simulink model "SPM_trial_5_simulink"  (R2023a)
settings: Solver=VariableStepAuto  StartTime=0.0  StopTime=500  RelTol=1e-3
values from neighbouring files (symbols this model uses):
  x_neg = 0:dx_n:del_n    [Generate_Amat_Electrolyte.m]
  x_pos = del_n+del_s:dx_p:del_n+del_s+del_p    [Generate_Amat_Electrolyte.m]
  x_sep = del_n:dx_s:del_n+del_s    [Generate_Amat_Electrolyte.m]
undefined symbols (not defined in the file or in its folder): CC, cs_init_n, cs_init_p, I, Iin, Ilim, Kaw, KI, nn, np, ns, sw, Vlim, Vmax
libraries: nesl_utility x16, fl_lib x4
settings Model: Creator=YASH PATHAK  LastModifiedBy=siegeljb
settings ModelReferenceCC: EnableRefExpFcnMdlSchedulingChecks=on

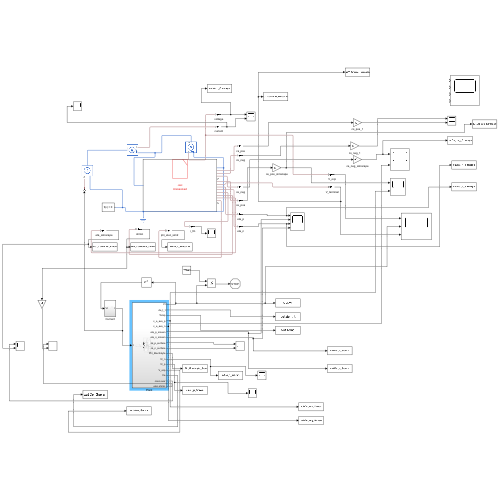
[thumbnail: Simulink's stored preview of the top-level diagram]
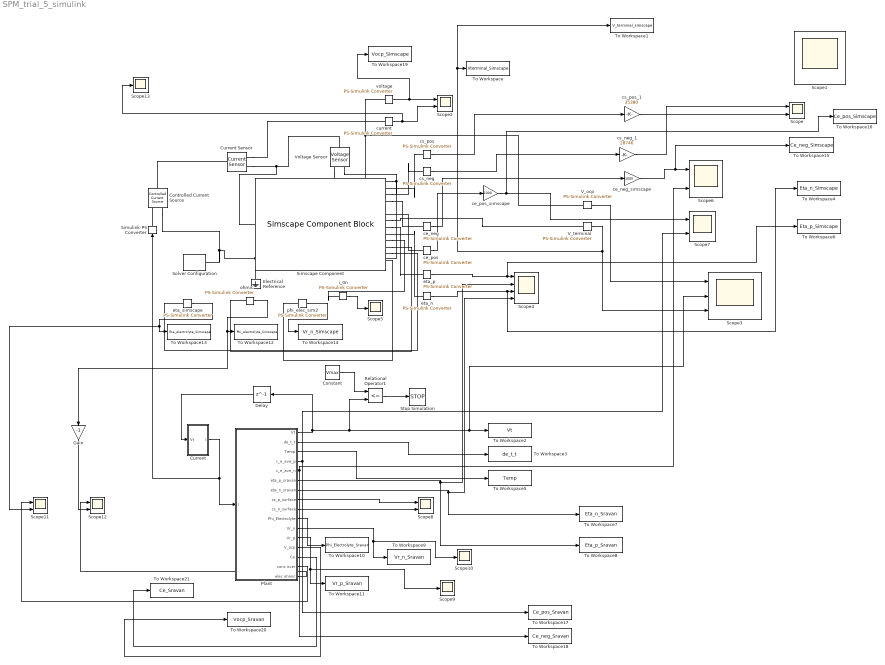
== system SPM_trial_5_simulink ==
  Constant : Constant  Value=Vmax
  Controlled Current Source : fl_lib/Electrical/Electrical Sources/Controlled Current Source
  Current : Subsystem
  Current Sensor : fl_lib/Electrical/Electrical Sensors/Current Sensor
  Delay : Delay  DelayLength=1
  Electrical Reference : fl_lib/Electrical/Electrical Elements/Electrical Reference
  Gain : Gain  Gain=-1
  Plant : Subsystem
  Relational Operator1 : RelationalOperator  Operator=<=  OutDataTypeStr=boolean  RndMeth=Simplest  InputSameDT=off
  Scope{,2,6..8,11..12} (7 alike) : Scope  NumInputPorts=2
  Scope1 : Scope  NumInputPorts=4
  Scope{5,9..10,13} (4 alike) : Scope
  Scope3 : Scope  NumInputPorts=3
  Scope4 : Scope  NumInputPorts=4
  Simscape Component : SimscapeComponentBlock  SourceFile=SPM_Trial_4_2  ComponentPath=SPM_Trial_4_2  ComponentVariants="[\"SPM_Trial_4_2\"]"  ComponentVariantNames="[\"SPM_Trial_4_2\"]"  ClassName=SPM_Trial_4_2  SchemaVersion=1  nr=50  nn=50  ns=25  np=50  Rp=3.5e-06 m  Rn=2.5e-06 m  Ds_p=8e-15 m^2/s  Ds_n=5e-15 m^2/s  D_e=5.35e-10 m^2/s  D_e1=5.35e-10  SOC_0=0.1  brugg=1.5  t_plus=0.38  tf=0.62  ce_init=1000 mol/m^3  ce_init_unitless=1000  kappa=1.3 S/m  k0_n=1.061e-6 / 96485  k0_p=4.824e-6 / 96485  kt_n=1 * 0.0250 V*m^2/A  kt_p=0 * 300e-4 V*m^2/A  x100_percent_n=0.8292  x0_percent_n=3.5506e-04  y0_percent_p=0.8941  y100_percent_p=0.0335  del_p=6.7e-05 m  del_n=6.2e-05 m  del_s=1.2e-05 m  del_p1=6.7e-05  del_n1=6.2e-05  del_s1=1.2e-05  cs_max_p=35380 mol/m^3  cs_max_p_unitless=35380  cs_max_n=28746 mol/m^3  cs_max_n_unitless=28746  epsilon_e_p=0.3  epsilon_e_n=0.3  epsilon_e_s=0.4  Active_Area=0.205 m^2  Faradays=96485 C/mol  T=273.15 + 25  R=8.3145  Cap_n=6.0272 C  Cap_p=5.8050 C  i_specify=off  i_priority=None  i=0 A  i_nominal_specify=off  i_nominal_unit=A  i_nominal_value=1  v_specify=off  v_priority=None  v=0 V  v_nominal_specify=off  v_nominal_unit=V  v_nominal_value=1  UP_specify=off  UP_priority=None  UP=0  UP_nominal_specify=off  UP_nominal_unit=1  UP_nominal_value=1  UN_specify=off  UN_priority=None  UN=0  UN_nominal_specify=off  UN_nominal_unit=1  UN_nominal_value=1  V_ocp_specify=off  V_ocp_priority=None  V_ocp=0  V_ocp_nominal_specify=off  V_ocp_nominal_unit=1  V_ocp_nominal_value=1  j_n_specify=off  j_n_priority=None  j_n=0  j_n_nominal_specify=off  j_n_nominal_unit=1  j_n_nominal_value=1  j_p_specify=off  j_p_priority=None  j_p=0  j_p_nominal_specify=off  j_p_nominal_unit=1  j_p_nominal_value=1  i0_p_specify=off  i0_p_priority=None  i0_p=0  i0_p_nominal_specify=off  i0_p_nominal_unit=1  i0_p_nominal_value=1  Vr_p_specify=off  Vr_p_priority=None  Vr_p=0  Vr_p_nominal_specify=off  Vr_p_nominal_unit=1  Vr_p_nominal_value=1  x_specify=off  x_priority=None  x=0  x_nominal_specify=off  x_nominal_unit=1  x_nominal_value=1  y_specify=off  y_priority=None  y=0  y_nominal_specify=off  y_nominal_unit=1  y_nominal_value=1
      settings: CopyFcn=simscape.engine.sli.internal.componentblockcallback(gcbh,'COPY')  PreCopyFcn=simscape.engine.sli.internal.componentblockcallback(gcbh,'PRECOPY')  PreDeleteFcn=simscape.engine.sli.internal.componentblockcallback(gcbh,'PREDELETE')  InternalSimscapePortConfiguration="{\"Bottom\":[],\"Left\":[{\"id\":\"p\",\"label\":\"+\",\"type\":\"foundation.electrical.electrical\"}],\"Right\":[{\"id\":\"n\",\"label\":\"-\",\"type\":\"foundation.electrical.electrical\"},{\"id\":\"cs_surf_p\",\"label\":\"cs_surf_p\",\"type\":\"output\"},{\"id\":\"cs_surf_n\",\"label\":\"cs_surf_n\",\"type\":\"output\"},{\"id\":\"ce_ave_n\",\"label\":\"ce_ave_n\",\"type\":\"output\"},{\"id\":\"ce_ave_s\",\"label\":\"ce_ave_s\",\"type\":\"output\"},{\"id\":\"ce_ave_p\",\"label\":\"ce_ave_p\",\"type\":\"output\"},{\"id\":\"V_terminal\",\"label\":\"V_terminal\",\"type\":\"output\"},{\"id\":\"eta_p\",\"label\":\"eta_p\",\"type\":\"output\"},{\"id\":\"eta_n\",\"label\":\"eta_n\",\"type\":\"output\"},{\"id\":\"i0_n\",\"label\":\"i0_n\",\"type\":\"output\"},{\"id\":\"phi_electrolyte\",\"label\":\"phi_electrolyte\",\"type\":\"output\"},{\"id\":\"eta_c\",\"label\":\"eta_c\",\"type\":\"output\"},{\"id\":\"Vr_n\",\"label\":\"Vr_n\",\"type\":\"output\"},{\"id\":\"ce_1\",\"label\":\"ce_1\",\"type\":\"output\"}],\"Top\":[]}"
      mask Type: Two-port electrical component
      mask Display: color('red');plot([0 1 1 0 0],[0 0 1 1 0]);plot([0.7,1],[1,0.7]);plot(-2,-1.75);plot(3, 1);disp('\n.ssc\nUnresolved')
  Simulink-PS Converter : nesl_utility/Simulink-PS Converter  PhysicalDomain=network_engine_domain  SubClassName=ps_input  LeftPortType=input  RightPortType=output  PseudoPeriodic=off  Frequencies=[]  NoiseDistribution=none  NoiseParameters=[]  Unit=1  AffineConversion=off  FilteringAndDerivatives=provide  SimscapeFilterOrder=1  InputFilterTimeConstant=0.001  UdotUserProvided=0
  Solver Configuration : nesl_utility/Solver Configuration  PhysicalDomain=network_engine_domain  SubClassName=solver  LeftPortType=input  RightPortType=generic  Tones=[]  Harmonics=[]  SimulateNoise=off  Profile=off  UseLocalSampling=off  EnableSwitchedLinearOptims=on  FrequencyDomain=off  UseCCode=off  RelTol=0.001  AbsTol=0.001  MinStep=1e-09  ToWorkspace=off  RevertToSquareIcSolve=off  NumHomotopyIterations=100  PhasorMode=off  PhasorModeNumHarmonics=1  ConsistencySolver=NEWTON_FTOL  IndexReductionMethod=DerivativeReplacement  DoDC=off  ResidualTolerance=1e-09  ConsistencyTolSource=GLOBAL  ConsistencyAbsTol=0.001  ConsistencyRelTol=0.001  ConsistencyTolFactor=0.001  UseLocalSolver=off  LocalSolverChoice=NE_BACKWARD_EULER_ADVANCER  ResolveIndetEquations=on  FunctionEvalNumThread=1  LocalSolverSampleTime=0.001  DoFixedCost=off  MaxNonlinIter=3  MaxModeIter=2  ComputeImpulses=off  ImpulseIterations=2  LinearAlgebra=auto  LinearAlgebraNumThread=0  EquationFormulation=NE_TIME_EF  DelaysMemoryBudget=1024  AutomaticFiltering=on  FilteringTimeConstant=0.001  PartitionStorageMethod=AS_NEEDED  PartitionMemoryBudget=1024  PartitionMethod=ROBUST
  Stop Simulation : Stop
  To Workspace : ToWorkspace  VariableName=Vterminal_Simscape  SaveFormat=Timeseries  SampleTime=-1
  To Workspace1 : ToWorkspace  VariableName=V_terminal_simscape  SampleTime=-1
  To Workspace10 : ToWorkspace  VariableName=Phi_Electrolyte_Sravan  SampleTime=-1
  To Workspace11 : ToWorkspace  VariableName=Vr_p_Sravan  SampleTime=-1
  To Workspace12 : ToWorkspace  VariableName=Phi_electrolyte_Simscape  SampleTime=-1
  To Workspace13 : ToWorkspace  VariableName=Eta_electrolyte_Simscape  SampleTime=-1
  To Workspace14 : ToWorkspace  VariableName=Vr_n_Simscape  SampleTime=-1
  To Workspace15 : ToWorkspace  VariableName=Ce_neg_Simscape  SampleTime=-1
  To Workspace16 : ToWorkspace  VariableName=Ce_pos_Simscape  SampleTime=-1
  To Workspace17 : ToWorkspace  VariableName=Ce_pos_Sravan  SampleTime=-1
  To Workspace18 : ToWorkspace  VariableName=Ce_neg_Sravan  SampleTime=-1
  To Workspace19 : ToWorkspace  VariableName=Vocp_Simscape  SampleTime=-1
  To Workspace2 : ToWorkspace  VariableName=Vt  SampleTime=1
  To Workspace20 : ToWorkspace  VariableName=Vocp_Sravan  SampleTime=-1
  To Workspace21 : ToWorkspace  VariableName=Ce_Sravan  SampleTime=-1
  To Workspace3 : ToWorkspace  VariableName=de_t_t  SampleTime=1
  To Workspace4 : ToWorkspace  VariableName=Eta_n_Simscape  SampleTime=-1
  To Workspace5 : ToWorkspace  VariableName=Temp  SampleTime=1
  To Workspace6 : ToWorkspace  VariableName=Eta_p_Simscape  SampleTime=-1
  To Workspace7 : ToWorkspace  VariableName=Eta_n_Sravan  SampleTime=-1
  To Workspace8 : ToWorkspace  VariableName=Eta_p_Sravan  SampleTime=-1
  To Workspace9 : ToWorkspace  VariableName=Vr_n_Sravan  SampleTime=-1
  V_ocp : nesl_utility/PS-Simulink Converter  PhysicalDomain=network_engine_domain  SubClassName=ps_output  LeftPortType=input  RightPortType=output  PseudoPeriodic=off  Frequencies=[]  VectorFormat=inherit  Unit=inherit  AffineConversion=off
  V_terminal : nesl_utility/PS-Simulink Converter  PhysicalDomain=network_engine_domain  SubClassName=ps_output  LeftPortType=input  RightPortType=output  PseudoPeriodic=off  Frequencies=[]  VectorFormat=inherit  Unit=inherit  AffineConversion=off
  Voltage Sensor : fl_lib/Electrical/Electrical Sensors/Voltage Sensor
  ce_neg : nesl_utility/PS-Simulink Converter  PhysicalDomain=network_engine_domain  SubClassName=ps_output  LeftPortType=input  RightPortType=output  PseudoPeriodic=off  Frequencies=[]  VectorFormat=inherit  Unit=inherit  AffineConversion=off
  ce_neg_simscape : Gain  Gain=1000
  ce_pos : nesl_utility/PS-Simulink Converter  PhysicalDomain=network_engine_domain  SubClassName=ps_output  LeftPortType=input  RightPortType=output  PseudoPeriodic=off  Frequencies=[]  VectorFormat=inherit  Unit=inherit  AffineConversion=off
  ce_pos_simscape : Gain  Gain=1000
  cs_neg : nesl_utility/PS-Simulink Converter  PhysicalDomain=network_engine_domain  SubClassName=ps_output  LeftPortType=input  RightPortType=output  PseudoPeriodic=off  Frequencies=[]  VectorFormat=inherit  Unit=inherit  AffineConversion=off
  cs_neg_1 : Gain  Gain=28746
  cs_pos : nesl_utility/PS-Simulink Converter  PhysicalDomain=network_engine_domain  SubClassName=ps_output  LeftPortType=input  RightPortType=output  PseudoPeriodic=off  Frequencies=[]  VectorFormat=inherit  Unit=inherit  AffineConversion=off
  cs_pos_1 : Gain  Gain=35380
  current : nesl_utility/PS-Simulink Converter  PhysicalDomain=network_engine_domain  SubClassName=ps_output  LeftPortType=input  RightPortType=output  PseudoPeriodic=off  Frequencies=[]  VectorFormat=inherit  Unit=inherit  AffineConversion=off
  eta_n : nesl_utility/PS-Simulink Converter  PhysicalDomain=network_engine_domain  SubClassName=ps_output  LeftPortType=input  RightPortType=output  PseudoPeriodic=off  Frequencies=[]  VectorFormat=inherit  Unit=inherit  AffineConversion=off
  eta_p : nesl_utility/PS-Simulink Converter  PhysicalDomain=network_engine_domain  SubClassName=ps_output  LeftPortType=input  RightPortType=output  PseudoPeriodic=off  Frequencies=[]  VectorFormat=inherit  Unit=inherit  AffineConversion=off
  eta_simscape : nesl_utility/PS-Simulink Converter  PhysicalDomain=network_engine_domain  SubClassName=ps_output  LeftPortType=input  RightPortType=output  PseudoPeriodic=off  Frequencies=[]  VectorFormat=inherit  Unit=inherit  AffineConversion=off
  i_0n : nesl_utility/PS-Simulink Converter  PhysicalDomain=network_engine_domain  SubClassName=ps_output  LeftPortType=input  RightPortType=output  PseudoPeriodic=off  Frequencies=[]  VectorFormat=inherit  Unit=inherit  AffineConversion=off
  ohmic : nesl_utility/PS-Simulink Converter  PhysicalDomain=network_engine_domain  SubClassName=ps_output  LeftPortType=input  RightPortType=output  PseudoPeriodic=off  Frequencies=[]  VectorFormat=inherit  Unit=inherit  AffineConversion=off
  phi_elec_sim2 : nesl_utility/PS-Simulink Converter  PhysicalDomain=network_engine_domain  SubClassName=ps_output  LeftPortType=input  RightPortType=output  PseudoPeriodic=off  Frequencies=[]  VectorFormat=inherit  Unit=inherit  AffineConversion=off
  voltage : nesl_utility/PS-Simulink Converter  PhysicalDomain=network_engine_domain  SubClassName=ps_output  LeftPortType=input  RightPortType=output  PseudoPeriodic=off  Frequencies=[]  VectorFormat=inherit  Unit=inherit  AffineConversion=off
  wires:
  ce_neg/1 -> ce_neg_simscape/1
  ce_pos/1 -> ce_pos_simscape/1
  voltage/1 -> To Workspace19/1, Scope2/1
  current/1 -> Scope13/1, Scope2/2
  V_terminal/1 -> To Workspace1/1, To Workspace/1, Scope3/3
  Plant/2(de_t_t) -> To Workspace3/1
  Delay/1 -> Current/1(Vt)
  Constant/1 -> Relational Operator1/1
  Plant/3(Temp) -> To Workspace5/1
  Plant/1(Vt) -> Delay/1, Relational Operator1/2, Scope3/2, To Workspace2/1
  Relational Operator1/1 -> Stop Simulation/1
  Current/1(I) -> Plant/1(I), Simulink-PS Converter/1
  eta_n/1 -> To Workspace4/1, Scope4/3
  eta_p/1 -> To Workspace6/1, Scope4/1
  i_0n/1 -> Scope5/1
  V_ocp/1 -> Scope3/1
  ce_pos_simscape/1 -> To Workspace16/1, Scope7/1
  ce_neg_simscape/1 -> To Workspace15/1, Scope6/1
  Plant/5(c_e_ave_n) -> To Workspace18/1, Scope6/2
  Plant/4(c_e_ave_p) -> To Workspace17/1, Scope7/2
  Plant/6(eta_p_sravan) -> To Workspace8/1, Scope4/2
  Plant/7(eta_n_sravan) -> To Workspace7/1, Scope4/4
  Plant/8(cs_p_surface) -> Scope8/1
  Plant/9(cs_n_surface) -> Scope8/2
  cs_pos_1/1 -> Scope/2
  cs_neg_1/1 -> Scope/1
  cs_pos/1 -> cs_pos_1/1
  cs_neg/1 -> cs_neg_1/1
  Plant/10(Phi_Electrolyte) -> To Workspace10/1
  Plant/11(Vr_n) -> To Workspace9/1, Scope10/1
  Plant/12(Vr_p) -> Scope9/1, To Workspace11/1
  ohmic/1 -> Gain/1, To Workspace12/1
  eta_simscape/1 -> Scope11/2, To Workspace13/1
  phi_elec_sim2/1 -> To Workspace14/1
  Plant/13(V_ocp) -> To Workspace20/1
  Plant/14(Ce) -> To Workspace21/1
  Plant/15(conc over) -> Scope11/1
  Plant/16(elec ohmic) -> Scope12/1
  Gain/1 -> Scope12/2
  connections:
  Simscape Component/RConn1 -- Voltage Sensor/RConn2 -- Electrical Reference/LConn1 -- Controlled Current Source/RConn2 -- Solver Configuration/RConn1
  Current Sensor/RConn2 -- Voltage Sensor/LConn1 -- Simscape Component/LConn1
  cs_pos/LConn1 -- Simscape Component/RConn2
  Simscape Component/RConn3 -- cs_neg/LConn1
  ce_pos/LConn1 -- Simscape Component/RConn6
  Simscape Component/RConn4 -- ce_neg/LConn1
  Voltage Sensor/RConn1 -- V_ocp/LConn1 -- voltage/LConn1
  Current Sensor/RConn1 -- current/LConn1
  Controlled Current Source/LConn1 -- Current Sensor/LConn1
  Simscape Component/RConn7 -- V_terminal/LConn1
  Simulink-PS Converter/RConn1 -- Controlled Current Source/RConn1
  eta_n/LConn1 -- Simscape Component/RConn9
  Simscape Component/RConn8 -- eta_p/LConn1
  Simscape Component/RConn10 -- i_0n/LConn1
  Simscape Component/RConn11 -- ohmic/LConn1
  Simscape Component/RConn12 -- eta_simscape/LConn1
  Simscape Component/RConn13 -- phi_elec_sim2/LConn1

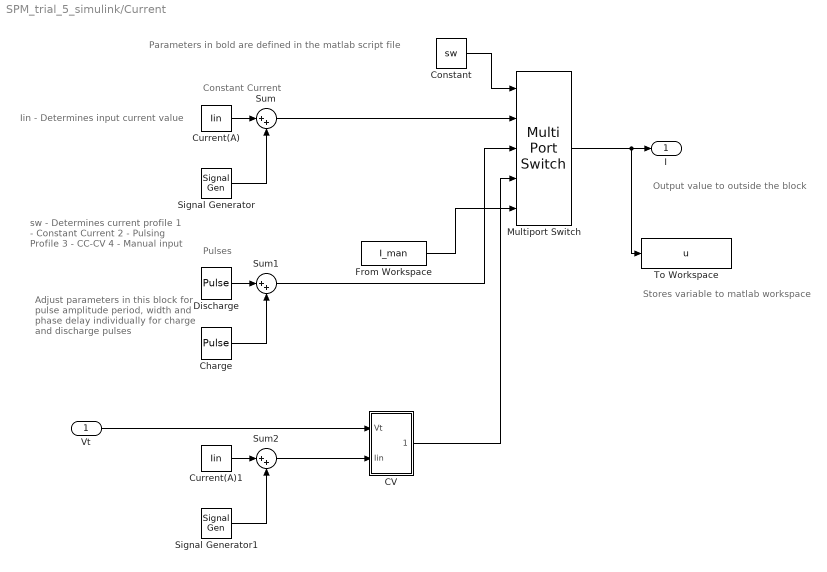
== system SPM_trial_5_simulink/Current ==
  note: Parameters in bold are defined in the matlab script file
  note: Adjust parameters in this block
      | for pulse amplitude period, width
      | and phase delay individually for
      | charge and discharge pulses
  note: Iin - Determines input current value
  note: Constant Current
  note: Pulses
  note: sw - Determines current profile
      | 1 - Constant Current
      | 2 - Pulsing Profile
      | 3 - CC-CV
      | 4 - Manual input
  note: Stores variable to matlab workspace
  note: Output value to outside the block
  Vt : Inport
  CV : Subsystem
  Charge : DiscretePulseGenerator  PulseType=Time based  Amplitude=-Iin/5  Period=100  PulseWidth=25  PhaseDelay=75
  Constant : Constant  Value=sw
  Current(A) : Constant  Value=Iin
  Current(A)1 : Constant  Value=Iin
  Discharge : DiscretePulseGenerator  PulseType=Time based  Amplitude=Iin  Period=100  PulseWidth=25  PhaseDelay=25
  From Workspace : FromWorkspace  VariableName=I_man
  Multiport Switch : MultiPortSwitch  Inputs=4  SaturateOnIntegerOverflow=off  InputSameDT=off
  Signal Generator : SignalGenerator  WaveForm=square  Amplitude=0
  Signal Generator1 : SignalGenerator  WaveForm=square  Amplitude=0  Frequency=0.1
  Sum : Sum  Inputs=|++
  Sum1 : Sum  Inputs=|++
  Sum2 : Sum  Inputs=|++
  To Workspace : ToWorkspace  VariableName=u  SampleTime=1
  I : Outport
  wires:
  Current(A)/1 -> Sum/1
  Discharge/1 -> Sum1/1
  Charge/1 -> Sum1/2
  Signal Generator/1 -> Sum/2
  Sum1/1 -> Multiport Switch/3
  Multiport Switch/1 -> To Workspace/1, I/1
  Sum/1 -> Multiport Switch/2
  Constant/1 -> Multiport Switch/1
  From Workspace/1 -> Multiport Switch/5
  Current(A)1/1 -> Sum2/1
  Sum2/1 -> CV/2(Iin)
  Signal Generator1/1 -> Sum2/2
  Vt/1 -> CV/1(Vt)
  CV/1(Iout) -> Multiport Switch/4

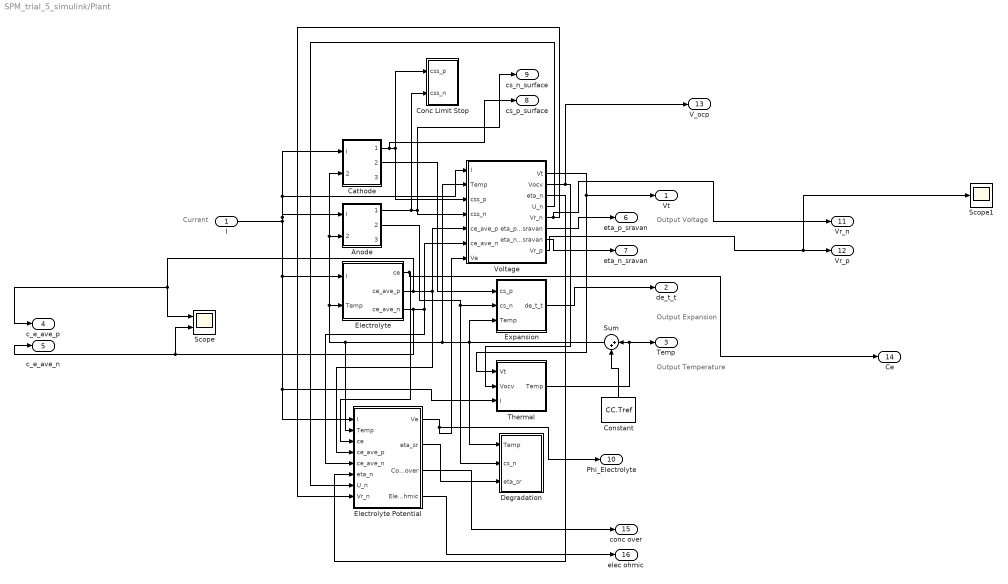
== system SPM_trial_5_simulink/Plant ==
  note: Output Voltage
  note: Output Expansion
  note: Output Temperature
  note: Current
  I : Inport
  Anode : Subsystem
  Cathode : Subsystem
  Conc Limit Stop : Subsystem
  Constant : Constant  Value=CC.Tref
  Degradation : Subsystem
  Electrolyte : Subsystem
  Electrolyte Potential : Subsystem
  Expansion : Subsystem
  Scope : Scope  NumInputPorts=2
  Scope1 : Scope
  Sum : Sum  Inputs=|++
  Thermal : Subsystem
  Voltage : Subsystem
  Vt : Outport
  de_t_t : Outport  Port=2
  Temp : Outport  Port=3
  c_e_ave_p : Outport  Port=4
  c_e_ave_n : Outport  Port=5
  eta_p_sravan : Outport  Port=6
  eta_n_sravan : Outport  Port=7
  cs_p_surface : Outport  Port=8
  cs_n_surface : Outport  Port=9
  Phi_Electrolyte : Outport  Port=10
  Vr_n : Outport  Port=11
  Vr_p : Outport  Port=12
  V_ocp : Outport  Port=13
  Ce : Outport  Port=14
  conc over : Outport  Port=15
  elec ohmic : Outport  Port=16
  wires:
  Cathode/2(cs_p) -> Expansion/1(cs_p)
  I/1 -> Cathode/1(I), Voltage/1(I), Anode/1(I), Electrolyte Potential/1(I), Thermal/3(I), Electrolyte/1(I)
  Anode/2(cs_n) -> Degradation/2(cs_n), Expansion/2(cs_n)
  Cathode/1(css_p) -> cs_p_surface/1, Voltage/3(css_p), Conc Limit Stop/1(css_p)
  Anode/1(css_n) -> cs_n_surface/1, Voltage/4(css_n), Conc Limit Stop/2(css_n)
  Voltage/1(Vt) -> Vt/1, Thermal/1(Vt)
  Sum/1 -> Degradation/1(Temp), Expansion/3(Temp), Voltage/2(Temp), Electrolyte/2(Temp), Cathode/2(Temp), Anode/2(Temp), Electrolyte Potential/2(Temp)
  Expansion/1(de_t_t) -> de_t_t/1
  Electrolyte/2(ce_ave_p) -> c_e_ave_p/1, Scope/1, Electrolyte Potential/4(ce_ave_p), Voltage/5(ce_ave_p)
  Electrolyte/3(ce_ave_n) -> c_e_ave_n/1, Scope/2, Electrolyte Potential/5(ce_ave_n), Voltage/6(ce_ave_n)
  Voltage/2(Vocv) -> V_ocp/1, Thermal/2(Vocv)
  Electrolyte/1(ce) -> Ce/1, Electrolyte Potential/3(ce)
  Voltage/3(eta_n) -> Electrolyte Potential/6(eta_n)
  Voltage/4(U_n) -> Electrolyte Potential/7(U_n)
  Electrolyte Potential/1(Ve) -> Voltage/7(Ve), Phi_Electrolyte/1
  Electrolyte Potential/2(eta_sr) -> Degradation/3(eta_sr)
  Thermal/1(Temp) -> Temp/1, Sum/1
  Constant/1 -> Sum/2
  Voltage/6(eta_p_sravan) -> eta_p_sravan/1
  Voltage/7(eta_n_sravan) -> eta_n_sravan/1
  Voltage/8(Vr_p) -> Scope1/1, Vr_p/1
  Voltage/5(Vr_n) -> Vr_n/1, Electrolyte Potential/8(Vr_n)
  Electrolyte Potential/3(Conc_over) -> conc over/1
  Electrolyte Potential/4(Elec_ohmic) -> elec ohmic/1

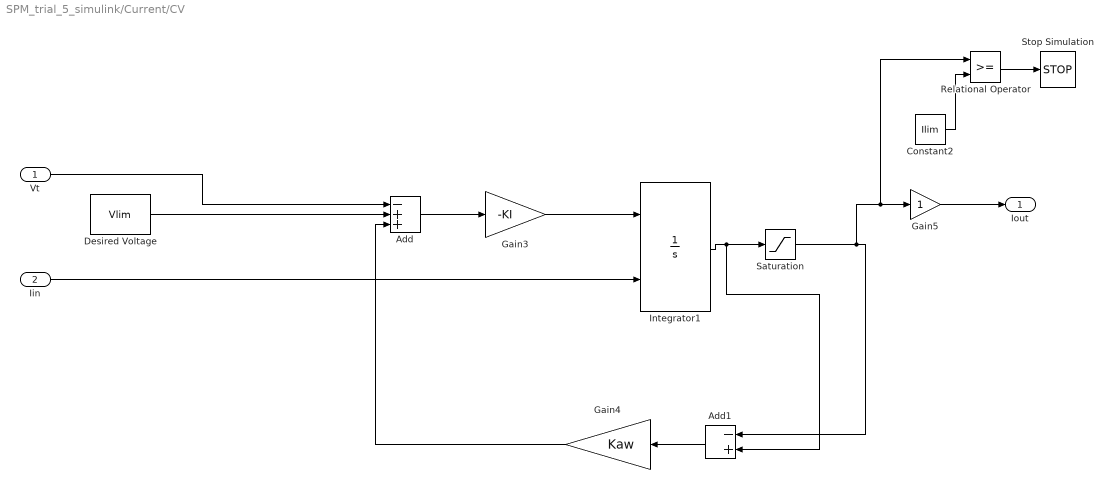
== system SPM_trial_5_simulink/Current/CV ==
  Vt : Inport
  Iin : Inport  Port=2
  Add : Sum  Inputs=-++
  Add1 : Sum  Inputs=-+
  Constant2 : Constant  Value=Ilim
  Desired Voltage : Constant  Value=Vlim
  Gain3 : Gain  Gain=-KI
  Gain4 : Gain  Gain=Kaw
  Gain5 : Gain
  Integrator1 : Integrator  InitialConditionSource=external  InitialCondition=I  UpperSaturationLimit=0  LowerSaturationLimit=-4.5
  Relational Operator : RelationalOperator  OutDataTypeStr=boolean  RndMeth=Simplest  InputSameDT=off
  Saturation : Saturate  UpperLimit=inf  LowerLimit=Iin
  Stop Simulation : Stop
  Iout : Outport
  wires:
  Vt/1 -> Add/1
  Iin/1 -> Integrator1/2
  Add/1 -> Gain3/1
  Add1/1 -> Gain4/1
  Gain4/1 -> Add/3
  Desired Voltage/1 -> Add/2
  Gain3/1 -> Integrator1/1
  Integrator1/1 -> Add1/2, Saturation/1
  Gain5/1 -> Iout/1
  Saturation/1 -> Relational Operator/1, Gain5/1, Add1/1
  Constant2/1 -> Relational Operator/2
  Relational Operator/1 -> Stop Simulation/1

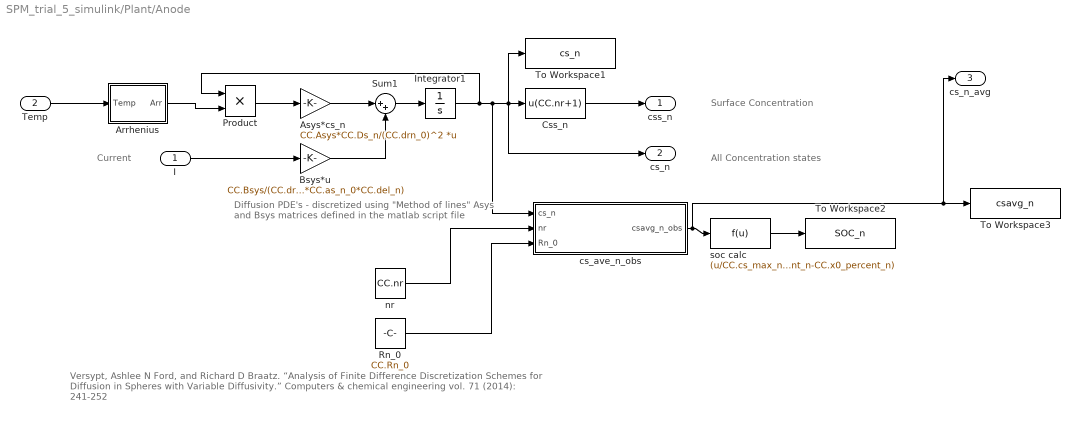
== system SPM_trial_5_simulink/Plant/Anode ==
  note: Current
  note: Surface Concentration
  note: All Concentration states
  note: Diffusion PDE's - discretized using "Method of lines"
      | Asys and Bsys matrices defined in the matlab script file
  note: Versypt, Ashlee N Ford, and Richard D Braatz. “Analysis of Finite Difference Discretization Schemes for Diffusion in Spheres with Variable Diffusivity.” Computers & chemical engineering vol. 71 (2014): 241-252
  I : Inport
  Temp : Inport  Port=2
  Arrhenius : Subsystem
  Asys*cs_n : Gain  Gain=CC.Asys*CC.Ds_n/(CC.drn_0)^2  Multiplication=Matrix(K*u)
  Bsys*u : Gain  Gain=CC.Bsys/(CC.drn_0*CC.F*CC.A*CC.as_n_0*CC.del_n)
  Css_n : Fcn  Expr=u(CC.nr+1)
  Integrator1 : Integrator  InitialCondition=cs_init_n*ones(CC.nr+1,1)
  Product : Product
  Rn_0 : Constant  Value=CC.Rn_0
  Sum1 : Sum  Inputs=|++
  To Workspace1 : ToWorkspace  VariableName=cs_n  SampleTime=1
  To Workspace2 : ToWorkspace  VariableName=SOC_n  SampleTime=1
  To Workspace3 : ToWorkspace  VariableName=csavg_n  SampleTime=1
  cs_ave_n_obs : MATLAB Function  TreatAsAtomicUnit=on
  nr : Constant  Value=CC.nr
  soc calc : Fcn  Expr=(u/CC.cs_max_n-CC.x0_percent_n)/(CC.x100_percent_n-CC.x0_percent_n)
  css_n : Outport
  cs_n : Outport  Port=2
  cs_n_avg : Outport  Port=3
  wires:
  Integrator1/1 -> Product/1, cs_ave_n_obs/1(cs_n), cs_n/1, Css_n/1, To Workspace1/1
  Asys*cs_n/1 -> Sum1/1
  Bsys*u/1 -> Sum1/2
  I/1 -> Bsys*u/1
  Sum1/1 -> Integrator1/1
  Css_n/1 -> css_n/1
  Rn_0/1 -> cs_ave_n_obs/3(Rn_0)
  nr/1 -> cs_ave_n_obs/2(nr)
  cs_ave_n_obs/1(csavg_n_obs) -> cs_n_avg/1, To Workspace3/1, soc calc/1
  soc calc/1 -> To Workspace2/1
  Arrhenius/1(Arr) -> Product/2
  Temp/1 -> Arrhenius/1(Temp)
  Product/1 -> Asys*cs_n/1

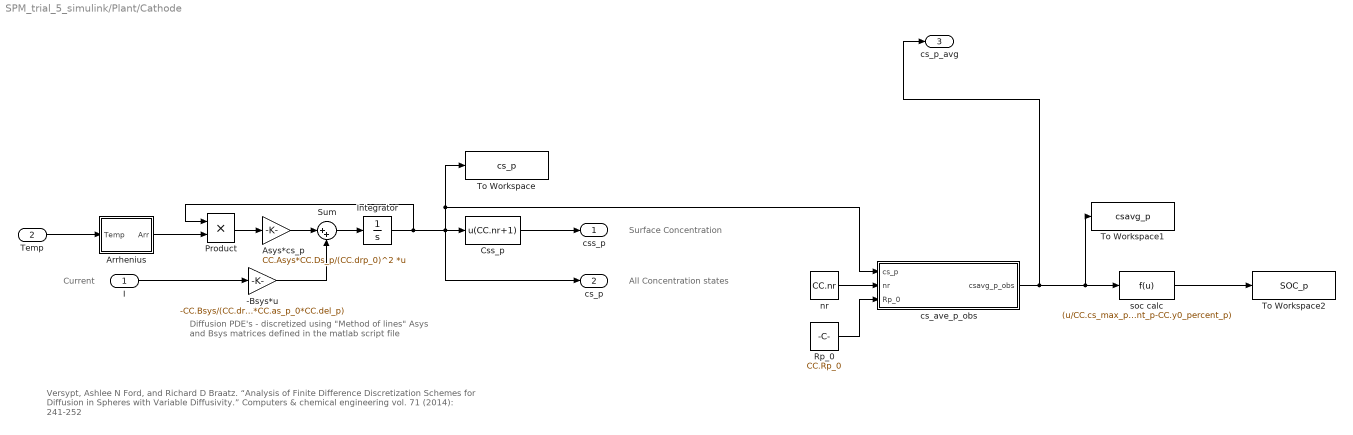
== system SPM_trial_5_simulink/Plant/Cathode ==
  note: Diffusion PDE's - discretized using "Method of lines"
      | Asys and Bsys matrices defined in the matlab script file
  note: All Concentration states
  note: Surface Concentration
  note: Current
  note: Versypt, Ashlee N Ford, and Richard D Braatz. “Analysis of Finite Difference Discretization Schemes for Diffusion in Spheres with Variable Diffusivity.” Computers & chemical engineering vol. 71 (2014): 241-252
  I : Inport
  Temp : Inport  Port=2
  -Bsys*u : Gain  Gain=-CC.Bsys/(CC.drp_0*CC.F*CC.A*CC.as_p_0*CC.del_p)
  Arrhenius : Subsystem
  Asys*cs_p : Gain  Gain=CC.Asys*CC.Ds_p/(CC.drp_0)^2  Multiplication=Matrix(K*u)
  Css_p : Fcn  Expr=u(CC.nr+1)
  Integrator : Integrator  InitialCondition=cs_init_p*ones(CC.nr+1,1)
  Product : Product
  Rp_0 : Constant  Value=CC.Rp_0
  Sum : Sum  Inputs=|++
  To Workspace : ToWorkspace  VariableName=cs_p  SampleTime=1
  To Workspace1 : ToWorkspace  VariableName=csavg_p  SampleTime=1
  To Workspace2 : ToWorkspace  VariableName=SOC_p  SampleTime=1
  cs_ave_p_obs : MATLAB Function  TreatAsAtomicUnit=on
  nr : Constant  Value=CC.nr
  soc calc : Fcn  Expr=(u/CC.cs_max_p-CC.y0_percent_p)/(CC.y100_percent_p-CC.y0_percent_p)
  css_p : Outport
  cs_p : Outport  Port=2
  cs_p_avg : Outport  Port=3
  wires:
  Arrhenius/1(Arr) -> Product/2
  Temp/1 -> Arrhenius/1(Temp)
  Product/1 -> Asys*cs_p/1
  Rp_0/1 -> cs_ave_p_obs/3(Rp_0)
  cs_ave_p_obs/1(csavg_p_obs) -> cs_p_avg/1, soc calc/1, To Workspace1/1
  Integrator/1 -> To Workspace/1, cs_ave_p_obs/1(cs_p), Css_p/1, cs_p/1, Product/1
  nr/1 -> cs_ave_p_obs/2(nr)
  soc calc/1 -> To Workspace2/1
  I/1 -> -Bsys*u/1
  Css_p/1 -> css_p/1
  Asys*cs_p/1 -> Sum/1
  Sum/1 -> Integrator/1
  -Bsys*u/1 -> Sum/2

== system SPM_trial_5_simulink/Plant/Conc Limit Stop ==
  css_p : Inport
  css_n : Inport  Port=2
  Constant1 : Constant  Value=0
  Constant2 : Constant  Value=CC.cs_max_p
  Constant3 : Constant  Value=0
  Constant4 : Constant  Value=CC.cs_max_n
  OR : Logic  Operator=OR  Inputs=4  IconShape=distinctive  AllPortsSameDT=off  OutDataTypeStr=boolean
  Relational Operator1 : RelationalOperator  Operator=<=  OutDataTypeStr=boolean  RndMeth=Simplest  InputSameDT=off
  Relational Operator2 : RelationalOperator  Operator=<=  OutDataTypeStr=boolean  RndMeth=Simplest  InputSameDT=off
  Relational Operator3 : RelationalOperator  OutDataTypeStr=boolean  RndMeth=Simplest  InputSameDT=off
  Relational Operator4 : RelationalOperator  OutDataTypeStr=boolean  RndMeth=Simplest  InputSameDT=off
  Stop Simulation1 : Stop
  wires:
  Constant3/1 -> Relational Operator3/1
  Relational Operator3/1 -> OR/3
  Relational Operator2/1 -> OR/4
  css_n/1 -> Relational Operator2/2, Relational Operator3/2
  Constant4/1 -> Relational Operator2/1
  Constant2/1 -> Relational Operator1/1
  Constant1/1 -> Relational Operator4/1
  OR/1 -> Stop Simulation1/1
  Relational Operator1/1 -> OR/2
  css_p/1 -> Relational Operator1/2, Relational Operator4/2
  Relational Operator4/1 -> OR/1

== system SPM_trial_5_simulink/Plant/Degradation ==
  Temp : Inport
  cs_n : Inport  Port=2
  eta_sr : Inport  Port=3
  Mechanical Stress : Subsystem
  Plating : Subsystem
  SEI : Subsystem
  wires:
  Temp/1 -> SEI/2(Temp), Plating/2(Temp)
  eta_sr/1 -> Plating/1(eta_sr), SEI/1(eta_sr)
  cs_n/1 -> Mechanical Stress/1(cs_n)

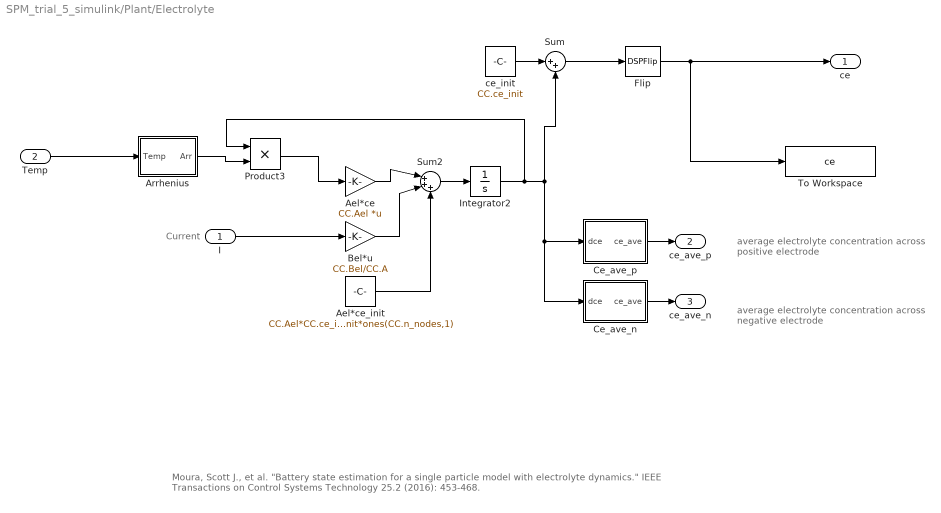
== system SPM_trial_5_simulink/Plant/Electrolyte ==
  note: Moura, Scott J., et al. "Battery state estimation for a single particle model with electrolyte dynamics." IEEE Transactions on Control Systems Technology 25.2 (2016): 453-468.
  note: Current
  note: average electrolyte concentration across
      | negative electrode
  note: average electrolyte concentration across
      | positive electrode
  I : Inport
  Temp : Inport  Port=2
  Ael*ce : Gain  Gain=CC.Ael  Multiplication=Matrix(K*u)
  Ael*ce_init : Constant  Value=CC.Ael*CC.ce_init*ones(CC.n_nodes,1)
  Arrhenius : Subsystem
  Bel*u : Gain  Gain=CC.Bel/CC.A
  Ce_ave_n : Subsystem
  Ce_ave_p : Subsystem
  Flip : DSPFlip
  Integrator2 : Integrator  InitialCondition=zeros(CC.n_nodes,1)
  Product3 : Product
  Sum : Sum  Inputs=|++
  Sum2 : Sum  Inputs=|+++
  To Workspace : ToWorkspace  VariableName=ce  SampleTime=1
  ce_init : Constant  Value=CC.ce_init
  ce : Outport
  ce_ave_p : Outport  Port=2
  ce_ave_n : Outport  Port=3
  wires:
  Temp/1 -> Arrhenius/1(Temp)
  Product3/1 -> Ael*ce/1
  Arrhenius/1(Arr) -> Product3/2
  Flip/1 -> To Workspace/1, ce/1
  I/1 -> Bel*u/1
  Ce_ave_n/1(ce_ave) -> ce_ave_n/1
  ce_init/1 -> Sum/1
  Sum/1 -> Flip/1
  Ce_ave_p/1(ce_ave) -> ce_ave_p/1
  Ael*ce/1 -> Sum2/1
  Bel*u/1 -> Sum2/2
  Sum2/1 -> Integrator2/1
  Ael*ce_init/1 -> Sum2/3
  Integrator2/1 -> Ce_ave_p/1(dce), Ce_ave_n/1(dce), Sum/2, Product3/1

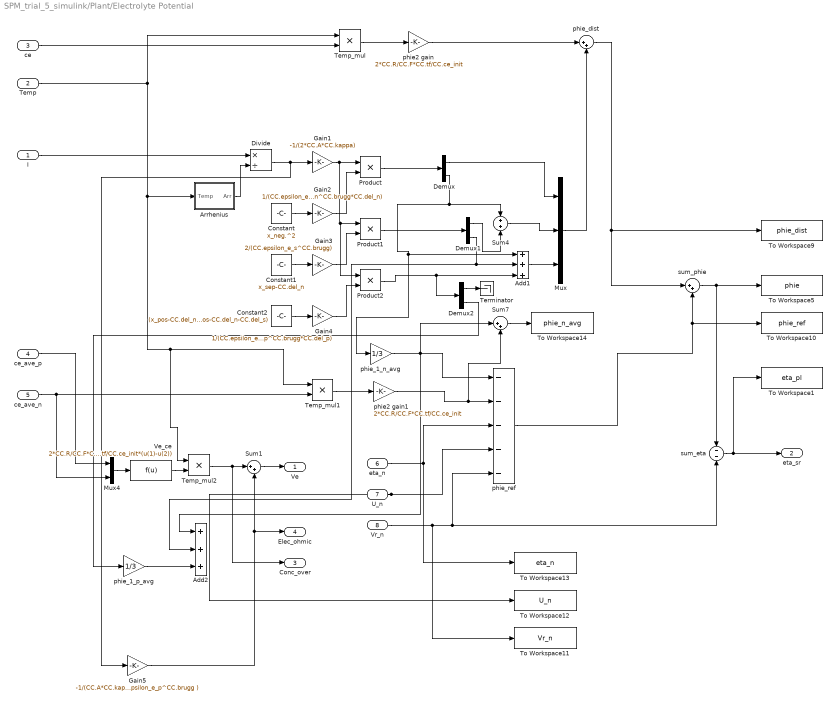
== system SPM_trial_5_simulink/Plant/Electrolyte Potential ==
  I : Inport
  Temp : Inport  Port=2
  ce : Inport  Port=3
  ce_ave_p : Inport  Port=4
  ce_ave_n : Inport  Port=5
  eta_n : Inport  Port=6
  U_n : Inport  Port=7
  Vr_n : Inport  Port=8
  Add1 : Sum  Inputs=+++
  Add2 : Sum  Inputs=+++
  Arrhenius : Subsystem
  Constant : Constant  Value=x_neg.^2
  Constant1 : Constant  Value=x_sep-CC.del_n
  Constant2 : Constant  Value=(x_pos-CC.del_n-CC.del_s).*(2*CC.del_t-x_pos-CC.del_n-CC.del_s)
  Demux : Demux  Outputs=[nn,1]
  Demux1 : Demux  Outputs=[ns,1]
  Demux2 : Demux  Outputs=[np,1]
  Divide : Product  Inputs=*/
  Gain1 : Gain  Gain=-1/(2*CC.A*CC.kappa)
  Gain2 : Gain  Gain=1/(CC.epsilon_e_n^CC.brugg*CC.del_n)
  Gain3 : Gain  Gain=2/(CC.epsilon_e_s^CC.brugg)
  Gain4 : Gain  Gain=1/(CC.epsilon_e_p^CC.brugg*CC.del_p)
  Gain5 : Gain  Gain=-1/(CC.A*CC.kappa)*(CC.del_n/3/CC.epsilon_e_n^CC.brugg+CC.del_s/CC.epsilon_e_s^CC.brugg+CC.del_p/3/CC.epsilon_e_p^CC.brugg )
  Mux : Mux  Inputs=3
  Mux4 : Mux  Inputs=2
  Product : Product
  Product1 : Product
  Product2 : Product
  Sum1 : Sum  Inputs=|++
  Sum4 : Sum
  Sum7 : Sum  Inputs=|++
  Temp_mul : Product
  Temp_mul1 : Product
  Temp_mul2 : Product
  Terminator : Terminator
  To Workspace1 : ToWorkspace  VariableName=eta_pl  SampleTime=1
  To Workspace10 : ToWorkspace  VariableName=phie_ref  SampleTime=1
  To Workspace11 : ToWorkspace  VariableName=Vr_n  SampleTime=1
  To Workspace12 : ToWorkspace  VariableName=U_n  SampleTime=1
  To Workspace13 : ToWorkspace  VariableName=eta_n  SampleTime=1
  To Workspace14 : ToWorkspace  VariableName=phie_n_avg  SampleTime=1
  To Workspace5 : ToWorkspace  VariableName=phie  SampleTime=1
  To Workspace9 : ToWorkspace  VariableName=phie_dist  SampleTime=1
  Ve_ce : Fcn  Expr=2*CC.R/CC.F*CC.tf/CC.ce_init*(u(1)-u(2))
  phie2 gain : Gain  Gain=2*CC.R/CC.F*CC.tf/CC.ce_init
  phie2 gain1 : Gain  Gain=2*CC.R/CC.F*CC.tf/CC.ce_init
  phie_1_n_avg : Gain  Gain=1/3
  phie_1_p_avg : Gain  Gain=1/3
  phie_dist : Sum  Inputs=|++
  phie_ref : Sum  Inputs=-----
  sum_eta : Sum  Inputs=--
  sum_phie : Sum  Inputs=|++
  Ve : Outport
  eta_sr : Outport  Port=2
  Conc_over : Outport  Port=3
  Elec_ohmic : Outport  Port=4
  wires:
  I/1 -> Divide/1
  ce_ave_n/1 -> Mux4/2, Temp_mul1/2
  ce/1 -> Temp_mul/2
  sum_eta/1 -> eta_sr/1, To Workspace1/1
  phie_ref/1 -> To Workspace10/1, sum_phie/2
  phie_1_n_avg/1 -> Add2/1, Sum7/1, phie_ref/1
  Temp/1 -> Temp_mul/1, Arrhenius/1(Temp), Temp_mul2/1, Temp_mul1/1
  Demux/1 -> Mux/1
  Gain1/1 -> Product2/1, Product1/1, Product/1
  Constant/1 -> Gain2/1
  Arrhenius/1(Arr) -> Divide/2
  Constant1/1 -> Gain3/1
  Gain4/1 -> Product2/2
  Product1/1 -> Demux1/1
  Mux/1 -> phie_dist/2
  Gain3/1 -> Product1/2
  Gain2/1 -> Product/2
  sum_phie/1 -> sum_eta/1, To Workspace5/1
  Temp_mul1/1 -> phie2 gain1/1
  phie2 gain/1 -> phie_dist/1
  Product/1 -> Demux/1
  phie2 gain1/1 -> Sum7/2, phie_ref/2
  Vr_n/1 -> phie_ref/5, sum_eta/2, To Workspace11/1
  Demux/2 -> Sum4/1, Add1/1, phie_1_n_avg/1
  eta_n/1 -> phie_ref/3, To Workspace13/1
  Temp_mul/1 -> phie2 gain/1
  phie_dist/1 -> To Workspace9/1, sum_phie/1
  Constant2/1 -> Gain4/1
  Product2/1 -> Demux2/1, Add1/3
  U_n/1 -> phie_ref/4, To Workspace12/1
  Divide/1 -> Gain5/1, Gain1/1
  Sum7/1 -> To Workspace14/1
  Mux4/1 -> Ve_ce/1
  ce_ave_p/1 -> Mux4/1
  Ve_ce/1 -> Temp_mul2/2
  Temp_mul2/1 -> Conc_over/1, Sum1/1
  Sum4/1 -> Mux/2
  Demux1/1 -> Sum4/2
  Add1/1 -> Mux/3
  Demux1/2 -> Add1/2, Add2/2
  Demux2/1 -> Terminator/1
  phie_1_p_avg/1 -> Add2/3
  Demux2/2 -> phie_1_p_avg/1
  Gain5/1 -> Elec_ohmic/1, Sum1/2
  Sum1/1 -> Ve/1

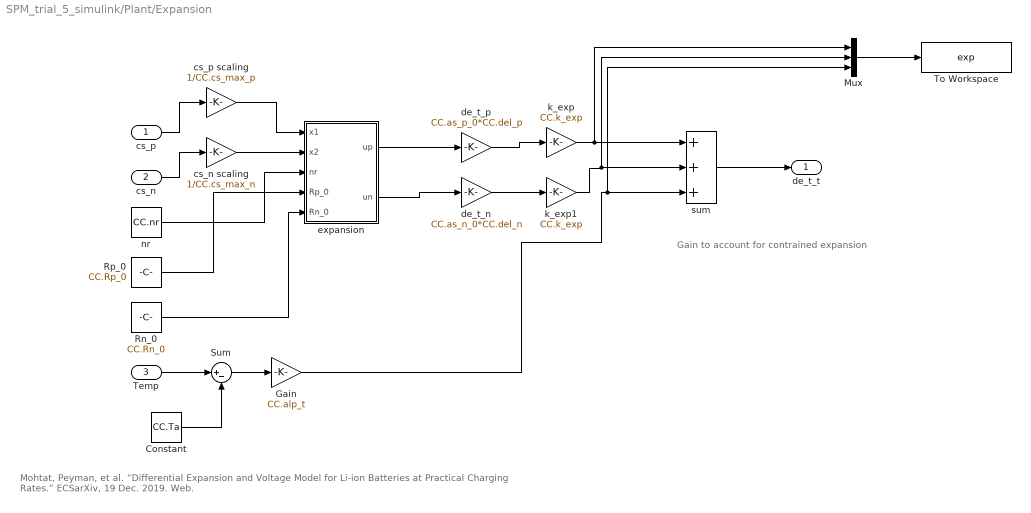
== system SPM_trial_5_simulink/Plant/Expansion ==
  note: Gain to account for contrained expansion
  note: Mohtat, Peyman, et al. “Differential Expansion and Voltage Model for Li-ion Batteries at Practical Charging Rates.” ECSarXiv, 19 Dec. 2019. Web.
  cs_p : Inport
  cs_n : Inport  Port=2
  Temp : Inport  Port=3
  Constant : Constant  Value=CC.Ta
  Gain : Gain  Gain=CC.alp_t
  Mux : Mux  Inputs=3
  Rn_0 : Constant  Value=CC.Rn_0
  Rp_0 : Constant  Value=CC.Rp_0
  Sum : Sum  Inputs=|+-
  To Workspace : ToWorkspace  VariableName=exp  SampleTime=1
  cs_n scaling : Gain  Gain=1/CC.cs_max_n
  cs_p scaling : Gain  Gain=1/CC.cs_max_p
  de_t_n : Gain  Gain=CC.as_n_0*CC.del_n
  de_t_p : Gain  Gain=CC.as_p_0*CC.del_p
  expansion : MATLAB Function  TreatAsAtomicUnit=on
  k_exp : Gain  Gain=CC.k_exp
  k_exp1 : Gain  Gain=CC.k_exp
  nr : Constant  Value=CC.nr
  sum : Sum  Inputs=+++
  de_t_t : Outport
  wires:
  de_t_n/1 -> k_exp1/1
  cs_n/1 -> cs_n scaling/1
  Rp_0/1 -> expansion/4(Rp_0)
  Rn_0/1 -> expansion/5(Rn_0)
  nr/1 -> expansion/3(nr)
  de_t_p/1 -> k_exp/1
  cs_p/1 -> cs_p scaling/1
  expansion/1(up) -> de_t_p/1
  expansion/2(un) -> de_t_n/1
  cs_p scaling/1 -> expansion/1(x1)
  cs_n scaling/1 -> expansion/2(x2)
  Temp/1 -> Sum/1
  Constant/1 -> Sum/2
  Sum/1 -> Gain/1
  Gain/1 -> Mux/3, sum/3
  sum/1 -> de_t_t/1
  Mux/1 -> To Workspace/1
  k_exp/1 -> Mux/1, sum/1
  k_exp1/1 -> Mux/2, sum/2

== system SPM_trial_5_simulink/Plant/Thermal ==
  note: Note: Ignoring entropic heating
  Vt : Inport
  Vocv : Inport  Port=2
  I : Inport  Port=3
  Abs : Abs  SaturateOnIntegerOverflow=off
  Constant : Constant  Value=CC.Ta
  Convection : Gain  Gain=CC.h
  Integrator : Integrator  InitialCondition=CC.T0
  Product : Product
  Scope : Scope
  Sum : Sum  Inputs=|+-
  Sum1 : Sum  Inputs=|-+
  Sum2 : Sum  Inputs=|+-
  Thermal Mass : Gain  Gain=1/CC.th_mass
  Temp : Outport
  wires:
  Sum1/1 -> Convection/1
  Abs/1 -> Sum2/1
  Integrator/1 -> Scope/1, Temp/1, Sum1/2
  Sum2/1 -> Thermal Mass/1
  Constant/1 -> Sum1/1
  Convection/1 -> Sum2/2
  Vt/1 -> Sum/1
  Vocv/1 -> Sum/2
  Sum/1 -> Product/1
  I/1 -> Product/2
  Product/1 -> Abs/1

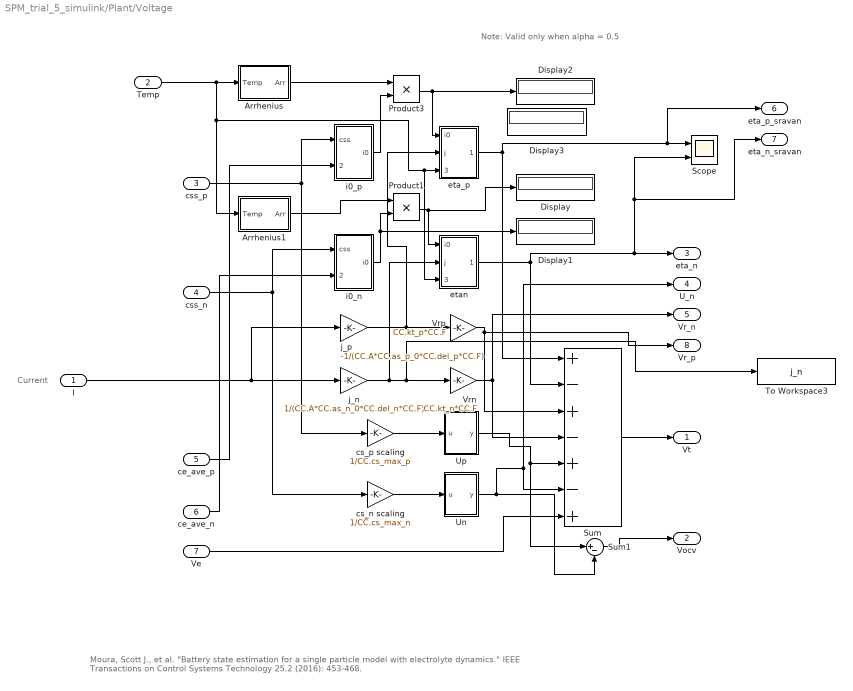
== system SPM_trial_5_simulink/Plant/Voltage ==
  note: Note: Valid only when alpha = 0.5
  note: Current
  note: Moura, Scott J., et al. "Battery state estimation for a single particle model with electrolyte dynamics." IEEE Transactions on Control Systems Technology 25.2 (2016): 453-468.
  I : Inport
  Temp : Inport  Port=2
  css_p : Inport  Port=3
  css_n : Inport  Port=4
  ce_ave_p : Inport  Port=5
  ce_ave_n : Inport  Port=6
  Ve : Inport  Port=7
  Arrhenius : Subsystem
  Arrhenius1 : Subsystem
  Display{,1..3} (4 alike) : Display
  Product1 : Product
  Product3 : Product
  Scope : Scope  NumInputPorts=2
  Sum : Sum  Inputs=+-+-+-+
  Sum1 : Sum  Inputs=|+-
  To Workspace3 : ToWorkspace  VariableName=j_n  SampleTime=1
  Un : MATLAB Function  TreatAsAtomicUnit=on
  Up : MATLAB Function  TreatAsAtomicUnit=on
  Vrn : Gain  Gain=CC.kt_n*CC.F
  Vrp : Gain  Gain=CC.kt_p*CC.F
  cs_n scaling : Gain  Gain=1/CC.cs_max_n
  cs_p scaling : Gain  Gain=1/CC.cs_max_p
  eta_p : Subsystem
  etan : Subsystem
  i0_n : Subsystem
  i0_p : Subsystem
  j_n : Gain  Gain=1/(CC.A*CC.as_n_0*CC.del_n*CC.F)
  j_p : Gain  Gain=-1/(CC.A*CC.as_p_0*CC.del_p*CC.F)
  Vt : Outport
  Vocv : Outport  Port=2
  eta_n : Outport  Port=3
  U_n : Outport  Port=4
  Vr_n : Outport  Port=5
  eta_p_sravan : Outport  Port=6
  eta_n_sravan : Outport  Port=7
  Vr_p : Outport  Port=8
  wires:
  j_n/1 -> etan/2(j), To Workspace3/1, Vrn/1
  j_p/1 -> Vrp/1, eta_p/2(j)
  eta_p/1(eta) -> eta_p_sravan/1, Scope/1, Sum/1
  etan/1(eta) -> Sum/2, eta_n_sravan/1, Scope/2, eta_n/1
  cs_n scaling/1 -> Un/1(u)
  i0_p/1(i0) -> Product3/2
  i0_n/1(i0) -> Display1/1, Product1/2
  cs_p scaling/1 -> Up/1(u)
  I/1 -> j_p/1, j_n/1
  css_p/1 -> cs_p scaling/1, i0_p/1(css)
  Up/1(y) -> Sum1/1, Sum/5
  css_n/1 -> cs_n scaling/1, i0_n/1(css)
  Un/1(y) -> Sum1/2, U_n/1, Sum/6
  Vrp/1 -> Vr_p/1, Sum/3
  ce_ave_p/1 -> i0_p/2(ce_ave)
  ce_ave_n/1 -> i0_n/2(ce_ave)
  Sum/1 -> Vt/1
  Sum1/1 -> Vocv/1
  Vrn/1 -> Vr_n/1, Sum/4
  Temp/1 -> Arrhenius/1(Temp), Arrhenius1/1(Temp), eta_p/3(Temp), etan/3(Temp)
  Product3/1 -> eta_p/1(i0), Display2/1
  Arrhenius1/1(Arr) -> Product1/1
  Ve/1 -> Sum/7
  Arrhenius/1(Arr) -> Product3/1
  Product1/1 -> etan/1(i0), Display/1

== system SPM_trial_5_simulink/Plant/Anode/Arrhenius ==
  Temp : Inport
  Constant : Constant  Value=1/CC.T
  Gain : Gain  Gain=CC.E_Ds_n/CC.R
  Math Function : Math
  Reciprocal : Product  Inputs=/
  Subtract : Sum  Inputs=+-
  Arr : Outport
  wires:
  Subtract/1 -> Gain/1
  Reciprocal/1 -> Subtract/2
  Constant/1 -> Subtract/1
  Math Function/1 -> Arr/1
  Temp/1 -> Reciprocal/1
  Gain/1 -> Math Function/1

== system SPM_trial_5_simulink/Plant/Cathode/Arrhenius ==
  Temp : Inport
  Constant : Constant  Value=1/CC.T
  Gain : Gain  Gain=CC.E_Ds_p/CC.R
  Math Function : Math
  Reciprocal : Product  Inputs=/
  Subtract : Sum  Inputs=+-
  Arr : Outport
  wires:
  Subtract/1 -> Gain/1
  Reciprocal/1 -> Subtract/2
  Constant/1 -> Subtract/1
  Math Function/1 -> Arr/1
  Temp/1 -> Reciprocal/1
  Gain/1 -> Math Function/1

== system SPM_trial_5_simulink/Plant/Degradation/Mechanical Stress ==
  cs_n : Inport
  Add : Sum
  Gain : Gain  Gain=1/3
  Gain1 : Gain  Gain=2/3
  Rn_1 : Constant  Value=CC.Rn_0
  To Workspace4 : ToWorkspace  VariableName=sigma_r  SampleTime=1
      settings: Save2DSignal=2-D array (concatenate along first dimension)
  To Workspace5 : ToWorkspace  VariableName=sigma_t  SampleTime=1
      settings: Save2DSignal=2-D array (concatenate along first dimension)
  To Workspace6 : ToWorkspace  VariableName=sigma_h  SampleTime=1
      settings: Save2DSignal=2-D array (concatenate along first dimension)
  const : Constant  Value=CC.Omega_nP*CC.E_nP/3/(1-CC.v_nP)
  nr1 : Constant  Value=CC.nr
  sigma : MATLAB Function  TreatAsAtomicUnit=on
  wires:
  sigma/2(sigma_t) -> Gain1/1, To Workspace5/1
  sigma/1(sigma_r) -> Gain/1, To Workspace4/1
  cs_n/1 -> sigma/1(cs_n)
  nr1/1 -> sigma/2(nr)
  Add/1 -> To Workspace6/1
  const/1 -> sigma/4(const)
  Gain/1 -> Add/1
  Gain1/1 -> Add/2
  Rn_1/1 -> sigma/3(Rn_0)

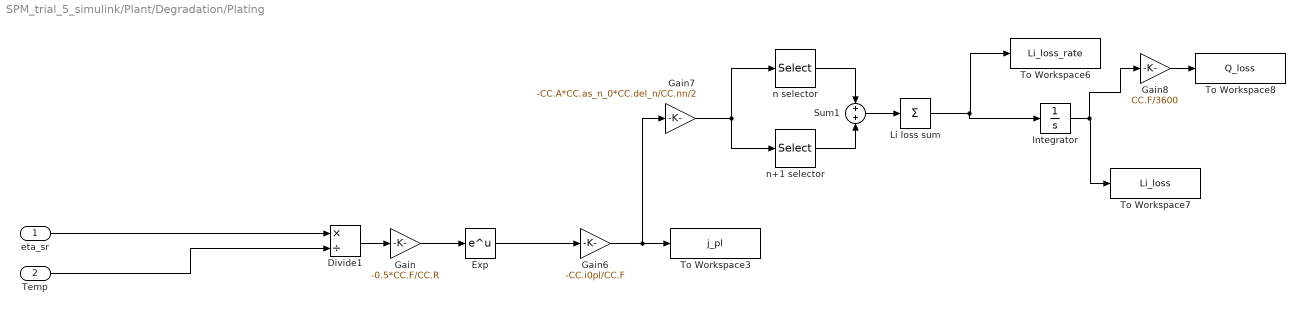
== system SPM_trial_5_simulink/Plant/Degradation/Plating ==
  eta_sr : Inport
  Temp : Inport  Port=2
  Divide1 : Product  Inputs=*/
  Exp : Math
  Gain : Gain  Gain=-0.5*CC.F/CC.R
  Gain6 : Gain  Gain=-CC.i0pl/CC.F
  Gain7 : Gain  Gain=-CC.A*CC.as_n_0*CC.del_n/CC.nn/2
  Gain8 : Gain  Gain=CC.F/3600
  Integrator : Integrator
  Li loss sum : Sum  Inputs=+
  Sum1 : Sum
  To Workspace3 : ToWorkspace  VariableName=j_pl  SampleTime=1
  To Workspace6 : ToWorkspace  VariableName=Li_loss_rate  SampleTime=1
  To Workspace7 : ToWorkspace  VariableName=Li_loss  SampleTime=1
  To Workspace8 : ToWorkspace  VariableName=Q_loss  SampleTime=1
  n selector : Selector  InputPortWidth=CC.n_nodes  IndexOptions=Index vector (dialog)  Indices=[1:CC.nn]  OutputSizes=1
  n+1 selector : Selector  InputPortWidth=CC.n_nodes  IndexOptions=Index vector (dialog)  Indices=[2:CC.nn+1]  OutputSizes=1
  wires:
  Gain6/1 -> Gain7/1, To Workspace3/1
  Gain7/1 -> n selector/1, n+1 selector/1
  Li loss sum/1 -> Integrator/1, To Workspace6/1
  Exp/1 -> Gain6/1
  Divide1/1 -> Gain/1
  Gain/1 -> Exp/1
  Sum1/1 -> Li loss sum/1
  Integrator/1 -> Gain8/1, To Workspace7/1
  Gain8/1 -> To Workspace8/1
  n selector/1 -> Sum1/1
  n+1 selector/1 -> Sum1/2
  eta_sr/1 -> Divide1/1
  Temp/1 -> Divide1/2

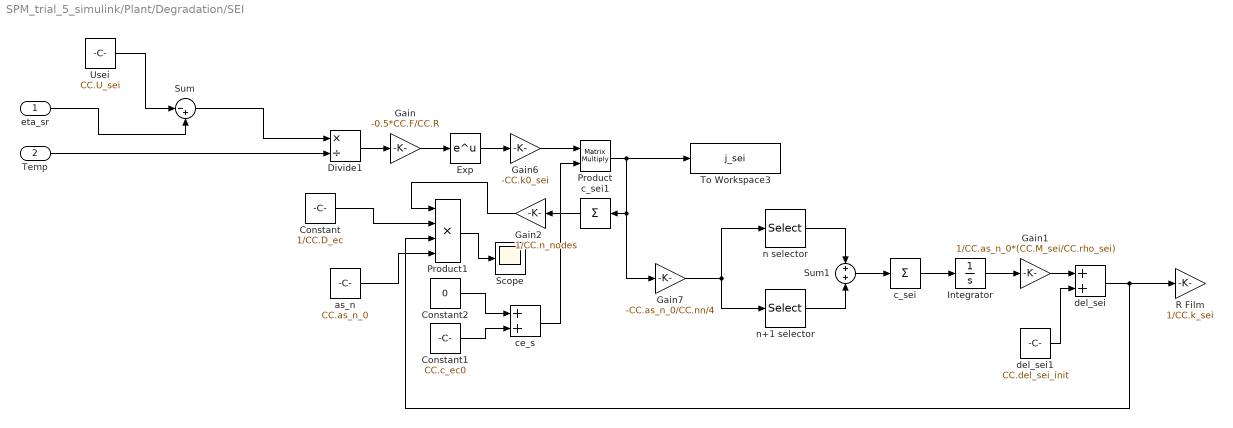
== system SPM_trial_5_simulink/Plant/Degradation/SEI ==
  eta_sr : Inport
  Temp : Inport  Port=2
  Constant : Constant  Value=1/CC.D_ec
  Constant1 : Constant  Value=CC.c_ec0
  Constant2 : Constant  Value=0
  Divide1 : Product  Inputs=*/
  Exp : Math
  Gain : Gain  Gain=-0.5*CC.F/CC.R
  Gain1 : Gain  Gain=1/CC.as_n_0*(CC.M_sei/CC.rho_sei)
  Gain2 : Gain  Gain=1/CC.n_nodes
  Gain6 : Gain  Gain=-CC.k0_sei
  Gain7 : Gain  Gain=-CC.as_n_0/CC.nn/4
  Integrator : Integrator
  Product : Product  Multiplication=Matrix(*)
  Product1 : Product  Inputs=4
  R Film : Gain  Gain=1/CC.k_sei
  Scope : Scope
  Sum : Sum  Inputs=|-+
  Sum1 : Sum
  To Workspace3 : ToWorkspace  VariableName=j_sei  SampleTime=1
  Usei : Constant  Value=CC.U_sei
  as_n : Constant  Value=CC.as_n_0
  c_sei : Sum  Inputs=+
  c_sei1 : Sum  Inputs=+
  ce_s : Sum
  del_sei : Sum
  del_sei1 : Constant  Value=CC.del_sei_init
  n selector : Selector  InputPortWidth=CC.n_nodes  IndexOptions=Index vector (dialog)  Indices=[1:CC.nn]  OutputSizes=1
  n+1 selector : Selector  InputPortWidth=CC.n_nodes  IndexOptions=Index vector (dialog)  Indices=[2:CC.nn+1]  OutputSizes=1
  wires:
  Exp/1 -> Gain6/1
  Divide1/1 -> Gain/1
  Gain/1 -> Exp/1
  eta_sr/1 -> Sum/2
  Usei/1 -> Sum/1
  Sum/1 -> Divide1/1
  Gain6/1 -> Product/1
  Product/1 -> To Workspace3/1, Gain7/1, c_sei1/1
  as_n/1 -> Product1/4
  del_sei/1 -> R Film/1, Product1/3
  Temp/1 -> Divide1/2
  Constant/1 -> Product1/2
  ce_s/1 -> Product/2
  n+1 selector/1 -> Sum1/2
  n selector/1 -> Sum1/1
  Sum1/1 -> c_sei/1
  Gain7/1 -> n selector/1, n+1 selector/1
  c_sei/1 -> Integrator/1
  Integrator/1 -> Gain1/1
  Gain1/1 -> del_sei/1
  del_sei1/1 -> del_sei/2
  c_sei1/1 -> Gain2/1
  Gain2/1 -> Product1/1
  Constant1/1 -> ce_s/2
  Constant2/1 -> ce_s/1
  Product1/1 -> Scope/1

== system SPM_trial_5_simulink/Plant/Electrolyte/Arrhenius ==
  Temp : Inport
  Constant : Constant  Value=1/CC.T
  Gain : Gain  Gain=CC.E_De/CC.R
  Math Function : Math
  Reciprocal : Product  Inputs=/
  Subtract : Sum  Inputs=+-
  Arr : Outport
  wires:
  Subtract/1 -> Gain/1
  Reciprocal/1 -> Subtract/2
  Constant/1 -> Subtract/1
  Math Function/1 -> Arr/1
  Temp/1 -> Reciprocal/1
  Gain/1 -> Math Function/1

== system SPM_trial_5_simulink/Plant/Electrolyte/Ce_ave_n ==
  dce : Inport
  ce_ave_p fcn : Fcn  Expr=u/(CC.nn+1)+CC.ce_init
  ce_n selector : Selector  InputPortWidth=CC.n_nodes  IndexOptions=Index vector (dialog)  Indices=[(np+ns)+1:(np+ns+nn)+1]  OutputSizes=1
  ce_n sum : Sum  Inputs=+
  ce_ave : Outport
  wires:
  ce_ave_p fcn/1 -> ce_ave/1
  dce/1 -> ce_n selector/1
  ce_n sum/1 -> ce_ave_p fcn/1
  ce_n selector/1 -> ce_n sum/1

== system SPM_trial_5_simulink/Plant/Electrolyte/Ce_ave_p ==
  dce : Inport
  ce_ave_p fcn : Fcn  Expr=u/(CC.np+1)+CC.ce_init
  ce_p selector : Selector  InputPortWidth=CC.n_nodes  IndexOptions=Index vector (dialog)  Indices=[1:CC.np+1]  OutputSizes=1
  ce_p sum : Sum  Inputs=+
  ce_ave : Outport
  wires:
  ce_ave_p fcn/1 -> ce_ave/1
  dce/1 -> ce_p selector/1
  ce_p sum/1 -> ce_ave_p fcn/1
  ce_p selector/1 -> ce_p sum/1

== system SPM_trial_5_simulink/Plant/Electrolyte Potential/Arrhenius ==
  Temp : Inport
  Constant : Constant  Value=1/CC.T
  Gain : Gain  Gain=CC.E_ke/CC.R
  Math Function : Math
  Reciprocal : Product  Inputs=/
  Subtract : Sum  Inputs=+-
  Arr : Outport
  wires:
  Subtract/1 -> Gain/1
  Reciprocal/1 -> Subtract/2
  Constant/1 -> Subtract/1
  Math Function/1 -> Arr/1
  Temp/1 -> Reciprocal/1
  Gain/1 -> Math Function/1

== system SPM_trial_5_simulink/Plant/Voltage/Arrhenius ==
  Temp : Inport
  Constant : Constant  Value=1/CC.T
  Gain : Gain  Gain=CC.E_r_p/CC.R
  Math Function : Math
  Reciprocal : Product  Inputs=/
  Subtract : Sum  Inputs=+-
  Arr : Outport
  wires:
  Subtract/1 -> Gain/1
  Reciprocal/1 -> Subtract/2
  Constant/1 -> Subtract/1
  Math Function/1 -> Arr/1
  Temp/1 -> Reciprocal/1
  Gain/1 -> Math Function/1

== system SPM_trial_5_simulink/Plant/Voltage/Arrhenius1 ==
  Temp : Inport
  Constant : Constant  Value=1/CC.T
  Gain : Gain  Gain=CC.E_r_n/CC.R
  Math Function : Math
  Reciprocal : Product  Inputs=/
  Subtract : Sum  Inputs=+-
  Arr : Outport
  wires:
  Subtract/1 -> Gain/1
  Reciprocal/1 -> Subtract/2
  Constant/1 -> Subtract/1
  Math Function/1 -> Arr/1
  Temp/1 -> Reciprocal/1
  Gain/1 -> Math Function/1

== system SPM_trial_5_simulink/Plant/Voltage/eta_p ==
  i0 : Inport
  j : Inport  Port=2
  Temp : Inport  Port=3
  Asinh : Trigonometry  Operator=asinh
  Fcn : Fcn  Expr=u(2)*CC.F/2/u(1)
  Gain : Gain  Gain=(CC.R/0.5/CC.F)
  Mux5 : Mux  Inputs=2
  Temp_mul : Product
  eta : Outport
  wires:
  Asinh/1 -> Temp_mul/2
  Fcn/1 -> Asinh/1
  i0/1 -> Mux5/1
  j/1 -> Mux5/2
  Mux5/1 -> Fcn/1
  Gain/1 -> eta/1
  Temp_mul/1 -> Gain/1
  Temp/1 -> Temp_mul/1

== system SPM_trial_5_simulink/Plant/Voltage/etan ==
  i0 : Inport
  j : Inport  Port=2
  Temp : Inport  Port=3
  Asinh : Trigonometry  Operator=asinh
  Fcn : Fcn  Expr=u(2)*CC.F/2/u(1)
  Gain : Gain  Gain=(CC.R/0.5/CC.F)
  Mux5 : Mux  Inputs=2
  Temp_mul : Product
  eta : Outport
  wires:
  Asinh/1 -> Temp_mul/2
  Fcn/1 -> Asinh/1
  i0/1 -> Mux5/1
  j/1 -> Mux5/2
  Mux5/1 -> Fcn/1
  Gain/1 -> eta/1
  Temp_mul/1 -> Gain/1
  Temp/1 -> Temp_mul/1

== system SPM_trial_5_simulink/Plant/Voltage/i0_n ==
  css : Inport
  ce_ave : Inport  Port=2
  Display : Display
  Display1 : Display
  Fcn : Fcn  Expr=u(2)*u(1)*(CC.cs_max_n-u(1))
  Gain : Gain  Gain=CC.k0_n.*CC.F
  Mux : Mux  Inputs=2
  Square Root : Sqrt
  i0 : Outport
  wires:
  Mux/1 -> Fcn/1
  ce_ave/1 -> Display/1, Mux/2
  Square Root/1 -> Gain/1
  Gain/1 -> i0/1
  css/1 -> Display1/1, Mux/1
  Fcn/1 -> Square Root/1

== system SPM_trial_5_simulink/Plant/Voltage/i0_p ==
  css : Inport
  ce_ave : Inport  Port=2
  Fcn : Fcn  Expr=u(2)*u(1)*(CC.cs_max_p-u(1))
  Gain : Gain  Gain=CC.k0_p.*CC.F
  Mux : Mux  Inputs=2
  Square Root : Sqrt
  i0 : Outport
  wires:
  Mux/1 -> Fcn/1
  ce_ave/1 -> Mux/2
  Square Root/1 -> Gain/1
  Gain/1 -> i0/1
  css/1 -> Mux/1
  Fcn/1 -> Square Root/1

== matlab function SPM_trial_5_simulink/Plant/Voltage/Un ==
  data: u input; y output
function y = fcn(u)

y = Un_0(u);

== matlab function SPM_trial_5_simulink/Plant/Voltage/Up ==
  data: u input; y output
function y = fcn(u)

y = Up_1(u);

== matlab function SPM_trial_5_simulink/Plant/Expansion/expansion ==
  data: x1 input; up output; x2 input; nr input; Rp_0 input; Rn_0 input; un output
function [up,un] = fcn(x1,x2,nr,Rp_0,Rn_0)
Rvec_p = 0:Rp_0/nr:Rp_0;
cube_p = ((Rvec_p(2:end)).^3-(Rvec_p(1:end-1)).^3);
Rvec_n = 0:Rn_0/nr:Rn_0;
cube_n = ((Rvec_n(2:end)).^3-(Rvec_n(1:end-1)).^3);

Mp = arrayfun(@ep_1, x1');
up = ((cube_p.*(Mp(1:end-1)+Mp(2:end))/2)*ones(nr,1))/(Rp_0^2)/3;
Mn = arrayfun(@en, x2');
un = ((cube_n.*(Mn(1:end-1)+Mn(2:end))/2)*ones(nr,1))/(Rn_0^2)/3;

end

== matlab function SPM_trial_5_simulink/Plant/Cathode/cs_ave_p_obs ==
  data: cs_p input; csavg_p_obs output; nr input; Rp_0 input
function csavg_p_obs = fcn(cs_p,nr,Rp_0)
cs_p = cs_p';
Rvec = 0:Rp_0/nr:Rp_0;
cube = ((Rvec(2:end)).^3-(Rvec(1:end-1)).^3);
muln = (cs_p(1:end-1)+cs_p(2:end))/2;
csavg_p_obs = ((cube.*muln)*ones(nr,1))/(Rp_0^3);

== matlab function SPM_trial_5_simulink/Plant/Anode/cs_ave_n_obs ==
  data: cs_n input; csavg_n_obs output; nr input; Rn_0 input
function csavg_n_obs = fcn(cs_n,nr,Rn_0)
cs_n = cs_n';
Rvec = 0:Rn_0/nr:Rn_0;
cube = ((Rvec(2:end)).^3-(Rvec(1:end-1)).^3);
muln = (cs_n(1:end-1)+cs_n(2:end))/2;
csavg_n_obs = ((cube.*muln)*ones(nr,1))/(Rn_0^3);

== matlab function SPM_trial_5_simulink/Plant/Degradation/Mechanical Stress/sigma ==
  data: cs_n input; sigma_r output; nr input [0..nr+1]; Rn_0 input; const input; sigma_t output
function [sigma_r,sigma_t] = fcn(cs_n,nr,Rn_0,const) %,sigma_r,sigma_t
cs_n = cs_n';
Rvec = 0:Rn_0/nr:Rn_0;
cube = ((Rvec(2:end)).^3-(Rvec(1:end-1)).^3);
muln = (cs_n(1:end-1)+cs_n(2:end))/2;
% csavg_n = ((cube.*muln)*ones(nr,1))/(Rn_0^3);
% csavg_n_obs = ((cube.*muln)*ones(nr,1))/(Rn_0^3);

sigma_r = zeros(size(cs_n'));
sigma_r(1) = (2*const)*(1/Rn_0^3*(1/3*(cube.*muln)*ones(nr,1))-1/3*cs_n(1));
sigma_t = zeros(size(cs_n'));
sigma_t(1) = (1*const)*(2/Rn_0^3*(1/3*(cube.*muln)*ones(nr,1))+1/3*cs_n(1)-cs_n(1));
for i=1:nr
    sigma_r(i+1) = (2*const)*(1/Rn_0^3*(1/3*(cube.*muln)*ones(nr,1))-1/(i/nr*Rn_0)^3*(1/3*(cube(1:i).*muln(1:i))*ones(i,1)));
    sigma_t(i+1) = (1*const)*(2/Rn_0^3*(1/3*(cube.*muln)*ones(nr,1))+1/(i/nr*Rn_0)^3*(1/3*(cube(1:i).*muln(1:i))*ones(i,1))-cs_n(i+1));
end

end
